simulink model "Silva_Simulink"  (R2024a)
settings: Solver=ode4  StartTime=0.0  StopTime=30  FixedStep=0.01  MaxStep=0.01  RelTol=1e-8  AbsTol=1e-8
values from neighbouring files (symbols this model uses):
  EA_0 = deg2rad([0 0 0]')    [Choi_SimulinkScript.m]    (also in SADS_UKF_Script.m = deg2rad([10 10 0]'); pointMassTest.m = [0 0 0]')
  J_0 = [1.815  -0.014 0.004 ... (first row only)    [Choi_SimulinkScript.m]    (also in Silva_SimulinkScript.m = [0.265 -0.014 -0.035; -0.014 0.246 -0.018; -0.035 -0.018 0.4; pointMassTest.m = diag([0.0226, 0.0257 0.0266]))
  kp = 0.5    [Silva_Matlab.m]    (also in Silva_Matlab_Implementation.m; Silva_SimulinkScript.m)
  m = 14.307    [Silva_Matlab.m]    (also in Silva_Matlab_Implementation.m; Silva_SimulinkScript.m; ukf.m)
  m_mmu = 2 * ((0.015*6) + (n*.236) + 0.177)    (= 2.894)    [Choi_SimulinkScript.m]    (also in Silva_Matlab.m = 0.7; Silva_Matlab_Implementation.m = 0.7; Silva_SimulinkScript.m = 0.7)
  omega_0 = [0 0.00 0.03]'    [Choi_SimulinkScript.m]    (also in SADS_UKF_Script.m = [0 0.00 0.00]'; Silva_SimulinkScript.m = [0 0 0.005]')
  q_0 = [0.99 -0.005 -0.063 -0.105]'    [Choi_SimulinkScript.m]    (also in SADS_UKF_Script.m = eul2quat(EA_0',"XYZ")'; Silva_SimulinkScript.m = [1 0 0 0]'; pointMassTest.m = [0 0 0 1]')
  r_b_0 = [-1 -3 -5]'*10^-3    [Silva_SimulinkScript.m]    (also in pointMassTest.m = [1 -0.9 -1.4]'.*1e-4)
  r_est_0 = [0 0 0]'    [Silva_SimulinkScript.m]
  Rcm = [y(8); y(9); y(10)]    [Silva_Matlab.m]    (also in Silva_Matlab_Implementation.m; eom_ukf.m = [0; 0; y(7)]; ukf.m = [0.1; -0.3; -5]*1e-3)
settings Model: Creator=cocmc  LastModifiedBy=cocmc

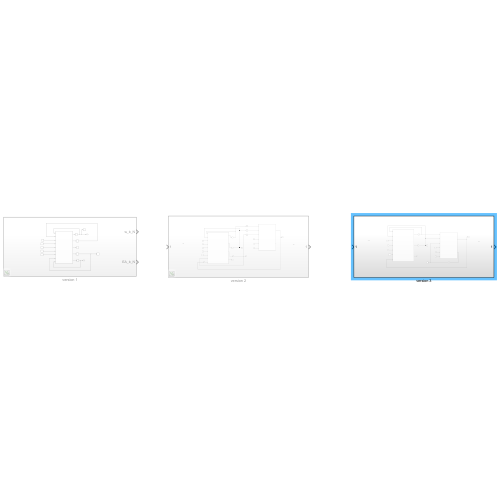
[thumbnail: Simulink's stored preview of the top-level diagram]
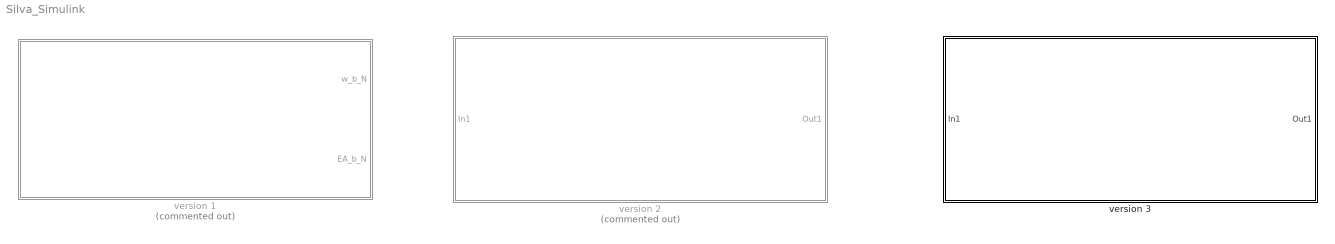
== system Silva_Simulink ==
  version 1 : Subsystem  Commented=on
  version 2 : Subsystem  Commented=on
  version 3 : Subsystem

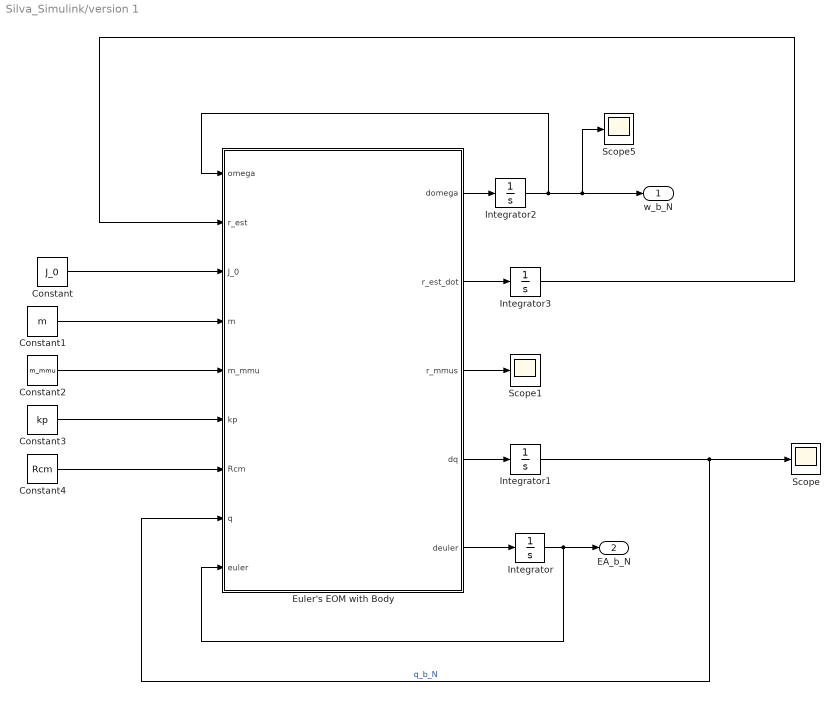
== system Silva_Simulink/version 1 ==
  Constant : Constant  Value=J_0
  Constant1 : Constant  Value=m
  Constant2 : Constant  Value=m_mmu
  Constant3 : Constant  Value=kp
  Constant4 : Constant  Value=Rcm
  Euler's EOM with Body : MATLAB Function  TreatAsAtomicUnit=on
  Integrator : Integrator  InitialCondition=EA_0
  Integrator1 : Integrator  InitialCondition=q_0
  Integrator2 : Integrator  InitialCondition=omega_0
  Integrator3 : Integrator  InitialCondition=r_est_0
  Scope : Scope
  Scope1 : Scope
  Scope5 : Scope
  w_b_N : Outport
  EA_b_N : Outport  Port=2
  wires:
  Constant1/1 -> Euler's EOM with Body/4(m)
  Euler's EOM with Body/1(domega) -> Integrator2/1
  Integrator2/1 -> Euler's EOM with Body/1(omega), Scope5/1, w_b_N/1
  Euler's EOM with Body/5(deuler) -> Integrator/1
  Integrator/1 -> EA_b_N/1, Euler's EOM with Body/9(euler)
  Euler's EOM with Body/4(dq) -> Integrator1/1
  Integrator1/1 -> Scope/1, Euler's EOM with Body/8(q)  "q_b_N"
  Euler's EOM with Body/2(r_est_dot) -> Integrator3/1
  Integrator3/1 -> Euler's EOM with Body/2(r_est)
  Constant/1 -> Euler's EOM with Body/3(J_0)
  Constant2/1 -> Euler's EOM with Body/5(m_mmu)
  Constant3/1 -> Euler's EOM with Body/6(kp)
  Constant4/1 -> Euler's EOM with Body/7(Rcm)
  Euler's EOM with Body/3(r_mmus) -> Scope1/1

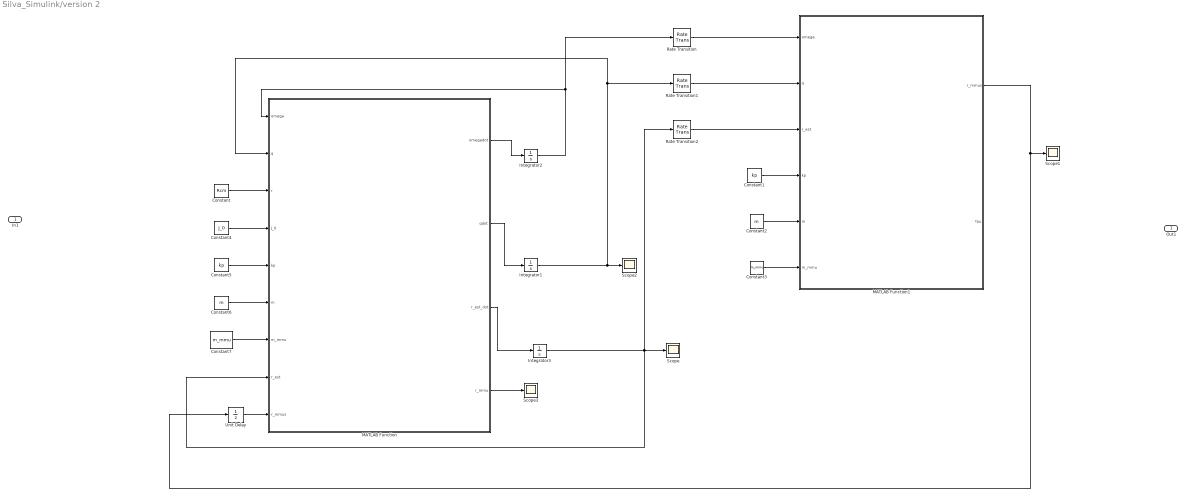
== system Silva_Simulink/version 2 ==
  In1 : Inport
  Constant : Constant  Value=Rcm
  Constant1 : Constant  Value=kp
  Constant2 : Constant  Value=m
  Constant3 : Constant  Value=m_mmu
  Constant4 : Constant  Value=J_0
  Constant5 : Constant  Value=kp
  Constant6 : Constant  Value=m
  Constant7 : Constant  Value=m_mmu
  Integrator1 : Integrator  InitialCondition=q_0
  Integrator2 : Integrator  InitialCondition=omega_0
  Integrator3 : Integrator  InitialCondition=r_est_0
  MATLAB Function : MATLAB Function  TreatAsAtomicUnit=on
  MATLAB Function1 : MATLAB Function  TreatAsAtomicUnit=on
  Rate Transition : RateTransition  InitialCondition=omega_0  OutPortSampleTime=control_sample
  Rate Transition1 : RateTransition  InitialCondition=q_0  OutPortSampleTime=control_sample
  Rate Transition2 : RateTransition  InitialCondition=r_est_0  OutPortSampleTime=control_sample
  Scope{,1..3} (4 alike) : Scope
  Unit Delay : UnitDelay  InitialCondition=[0 0 0]'  SampleTime=-1  HasFrameUpgradeWarning=on
  Out1 : Outport
  wires:
  MATLAB Function/1(omegadot) -> Integrator2/1
  MATLAB Function/2(qdot) -> Integrator1/1
  Integrator1/1 -> MATLAB Function/2(q), Rate Transition1/1, Scope2/1
  Integrator2/1 -> Rate Transition/1, MATLAB Function/1(omega)
  MATLAB Function/3(r_est_dot) -> Integrator3/1
  Integrator3/1 -> Rate Transition2/1, Scope/1, MATLAB Function/8(r_est)
  Constant/1 -> MATLAB Function/3(r)
  Constant1/1 -> MATLAB Function1/4(kp)
  MATLAB Function1/1(r_mmus) -> Unit Delay/1, Scope1/1
  Rate Transition/1 -> MATLAB Function1/1(omega)
  Rate Transition1/1 -> MATLAB Function1/2(q)
  Rate Transition2/1 -> MATLAB Function1/3(r_est)
  Unit Delay/1 -> MATLAB Function/9(r_mmus)
  Constant2/1 -> MATLAB Function1/5(m)
  Constant3/1 -> MATLAB Function1/6(m_mmu)
  Constant4/1 -> MATLAB Function/4(J_0)
  Constant5/1 -> MATLAB Function/5(kp)
  Constant6/1 -> MATLAB Function/6(m)
  Constant7/1 -> MATLAB Function/7(m_mmu)
  MATLAB Function/4(r_mmu) -> Scope3/1

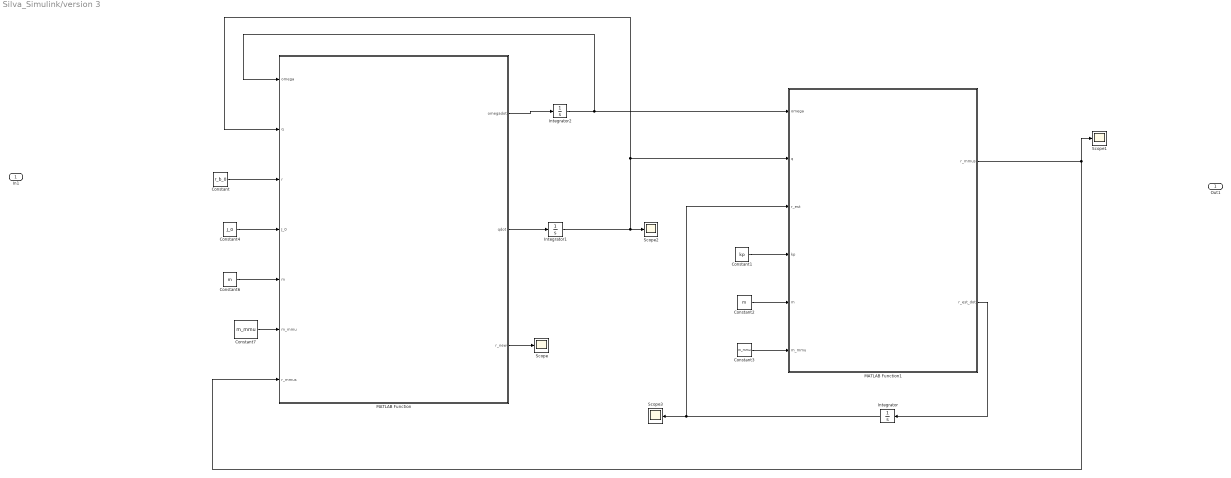
== system Silva_Simulink/version 3 ==
  In1 : Inport
  Constant : Constant  Value=r_b_0
  Constant1 : Constant  Value=kp
  Constant2 : Constant  Value=m
  Constant3 : Constant  Value=m_mmu
  Constant4 : Constant  Value=J_0
  Constant6 : Constant  Value=m
  Constant7 : Constant  Value=m_mmu
  Integrator : Integrator  InitialCondition=r_est_0
  Integrator1 : Integrator  InitialCondition=q_0
  Integrator2 : Integrator  InitialCondition=omega_0
  MATLAB Function : MATLAB Function  TreatAsAtomicUnit=on
  MATLAB Function1 : MATLAB Function  TreatAsAtomicUnit=on
  Scope{,1..3} (4 alike) : Scope
  Out1 : Outport
  wires:
  MATLAB Function/1(omegadot) -> Integrator2/1
  MATLAB Function/2(qdot) -> Integrator1/1
  Constant/1 -> MATLAB Function/3(r)
  Constant1/1 -> MATLAB Function1/4(kp)
  Constant2/1 -> MATLAB Function1/5(m)
  Constant3/1 -> MATLAB Function1/6(m_mmu)
  Constant4/1 -> MATLAB Function/4(J_0)
  Constant6/1 -> MATLAB Function/5(m)
  Constant7/1 -> MATLAB Function/6(m_mmu)
  MATLAB Function1/2(r_est_dot) -> Integrator/1
  Integrator/1 -> Scope3/1, MATLAB Function1/3(r_est)
  MATLAB Function/3(r_new) -> Scope/1
  MATLAB Function1/1(r_mmus) -> MATLAB Function/7(r_mmus), Scope1/1
  Integrator2/1 -> MATLAB Function1/1(omega), MATLAB Function/1(omega)
  Integrator1/1 -> MATLAB Function1/2(q), MATLAB Function/2(q), Scope2/1

== matlab function Silva_Simulink/version 3/MATLAB Function ==
  data: omega input; q input; r input; J_0 input; m input; m_mmu input; r_mmus input; omegadot output; qdot output; r_new output
function [omegadot, qdot,r_new] = fcn(omega,q,r,J_0,m,m_mmu,r_mmus)
% Equations of motion developed in the work of Chesi.

g = 9.81; % 


% Quaternion rates
qdot = 0.5*[0 -omega(1) -omega(2) -omega(3);
             omega(1) 0 omega(3) -omega(2);
             omega(2) -omega(3) 0 omega(1);
             omega(3) omega(2) -omega(1) 0]*q;

% Gravity vector in body-frame
Rbi = [2*q(1)^2-1+2*q(2)^2 2*q(2)*q(3)-2*q(1)*q(4) 2*q(2)*q(4)+2*q(1)*q(3);
       2*q(2)*q(3)+2*q(1)*q(4) 2*q(1)^2-1+2*q(3)^2 2*q(3)*q(4)-2*q(1)*q(2);
       2*q(2)*q(4)-2*q(1)*q(3) 2*q(3)*q(4)+2*q(1)*q(2) 2*q(1)^2-1+2*q(4)^2];

g_b = Rbi' * [0; 0; -9.81];

MMUx = [r_mmus(1); -0.22; 0];
MMUy = [0.22; r_mmus(2); 0];
MMUz = [-0.22; 0; r_mmus(3)];


Jaug = [m*(r(2)^2+r(3)^2) -m*r(1)*r(2) -m*r(1)*r(3);
        -m*r(1)*r(2) m*(r(1)^2+r(3)^2) -m*r(2)*r(3);
        -m*r(1)*r(3) -m*r(2)*r(3) m*(r(1)^2+r(2)^2)];

J = J_0 + Jaug;

% Update of inertia tensor
MMUxCross = [0 -MMUx(3) MMUx(2);
             MMUx(3) 0 -MMUx(1);
             -MMUx(2) MMUx(1) 0];

MMUyCross = [0 -MMUy(3) MMUy(2);
             MMUy(3) 0 -MMUy(1);
             -MMUy(2) MMUy(1) 0];

MMUzCross = [0 -MMUz(3) MMUz(2);
             MMUz(3) 0 -MMUz(1);
             -MMUz(2) MMUz(1) 0];

J = J - m_mmu * (MMUxCross*MMUxCross + MMUyCross*MMUyCross + MMUzCross*MMUzCross);

u = [1 0 0; % column vectors that each mass slides along
     0 1 0;
     0 0 1];



sum = zeros(size(u,2), 1);
for i = 1:size(u,2)
    sum = sum + m_mmu*r_mmus(i)*u(:,i);
end

r_new = r + (1/m).*sum;


tau = m_mmu * cross(r_mmus,g_b);
tau = 0;

r = r_new;

%% Dynamics equation
omegadot=J\(-cross(omega,J*omega)+cross(r,g_b*m)+tau);

== matlab function Silva_Simulink/version 3/MATLAB Function1 ==
  data: omega input; q input; r_mmus output; r_est_dot output; r_est input; kp input; m input; m_mmu input
function [r_mmus,r_est_dot] = fcn(omega,q,r_est,kp,m,m_mmu)
    Rbi = [2*q(1)^2-1+2*q(2)^2 2*q(2)*q(3)-2*q(1)*q(4) 2*q(2)*q(4)+2*q(1)*q(3);
           2*q(2)*q(3)+2*q(1)*q(4) 2*q(1)^2-1+2*q(3)^2 2*q(3)*q(4)-2*q(1)*q(2);
           2*q(2)*q(4)-2*q(1)*q(3) 2*q(3)*q(4)+2*q(1)*q(2) 2*q(1)^2-1+2*q(4)^2];

    g_b = Rbi' * [0; 0; -9.81];


    % Projection operator
    P = eye(3) - g_b*g_b'/norm(g_b)^2;
    omega_p = P*omega;
    gbcross = [0 -g_b(3) g_b(2);
               g_b(3) 0 -g_b(1);
              -g_b(2) g_b(1) 0];
    
    Phi = -m*gbcross;
    tau = -Phi*r_est-kp*omega_p;
    
    r_mmus = gbcross*tau/(norm(g_b)^2*m_mmu);


    % Adaptive control law for the estimated unbalance vector
    r_est_dot = Phi'*omega;

== matlab function Silva_Simulink/version 2/MATLAB Function1 ==
  data: omega input; q input; r_mmus output; r_est input; kp input; m input; m_mmu input; tau output
function [r_mmus,tau] = fcn(omega,q,r_est,kp,m,m_mmu)
    Rbi = [2*q(1)^2-1+2*q(2)^2 2*q(2)*q(3)-2*q(1)*q(4) 2*q(2)*q(4)+2*q(1)*q(3);
           2*q(2)*q(3)+2*q(1)*q(4) 2*q(1)^2-1+2*q(3)^2 2*q(3)*q(4)-2*q(1)*q(2);
           2*q(2)*q(4)-2*q(1)*q(3) 2*q(3)*q(4)+2*q(1)*q(2) 2*q(1)^2-1+2*q(4)^2];

    gb = Rbi' * [0; 0; -9.81];
    gbcross = [0 -gb(3) gb(2);
               gb(3) 0 -gb(1);
              -gb(2) gb(1) 0];

    % control torque at end of time step
    
    Phi = -m*gbcross;
    P = eye(3) - gb*gb'/norm(gb)^2;
    omegap = P*omega;
    tau = -Phi*r_est-kp*omegap;

    % Determine the new r_mmus vector. Dynamics of the MMUs are not considered,
    % which means r_mmus changes instantaneously
    r_mmus = gbcross*tau/(norm(gb)^2*m_mmu);

== matlab function Silva_Simulink/version 2/MATLAB Function ==
  data: omega input; q input; r input; J_0 input; kp input; m input; m_mmu input; r_est input; r_mmus input; omegadot output; qdot output; r_est_dot output; r_mmu output
function [omegadot, qdot, r_est_dot,r_mmu] = fcn(omega,q,r,J_0,kp,m,m_mmu,r_est,r_mmus)
% Equations of motion developed in the work of Chesi.

g = 9.81; % 


% Quaternion rates
qdot = 0.5*[0 -omega(1) -omega(2) -omega(3);
             omega(1) 0 omega(3) -omega(2);
             omega(2) -omega(3) 0 omega(1);
             omega(3) omega(2) -omega(1) 0]*q;

% Gravity vector in body-frame
Rbi = [2*q(1)^2-1+2*q(2)^2 2*q(2)*q(3)-2*q(1)*q(4) 2*q(2)*q(4)+2*q(1)*q(3);
       2*q(2)*q(3)+2*q(1)*q(4) 2*q(1)^2-1+2*q(3)^2 2*q(3)*q(4)-2*q(1)*q(2);
       2*q(2)*q(4)-2*q(1)*q(3) 2*q(3)*q(4)+2*q(1)*q(2) 2*q(1)^2-1+2*q(4)^2];

g_b = Rbi' * [0; 0; -g];

% Projection operator
P = eye(3) - g_b*g_b'/norm(g_b)^2;
omega_p = P*omega;
gbcross = [0 -g_b(3) g_b(2);
           g_b(3) 0 -g_b(1);
          -g_b(2) g_b(1) 0];

Phi = -m*gbcross;
tau = -Phi*r_est-kp*omega_p;

r_mmu = gbcross*tau/(norm(g_b)^2*m_mmu);
tau = m_mmu * cross(r_mmu,g_b);

% Adaptive control law for the estimated unbalance vector
r_est_dot = Phi'*omega;

MMUx = [r_mmus(1); -0.22; 0];
MMUy = [0.22; r_mmus(2); 0];
MMUz = [-0.22; 0; r_mmus(3)];


Jaug = [m*(r(2)^2+r(3)^2) -m*r(1)*r(2) -m*r(1)*r(3);
        -m*r(1)*r(2) m*(r(1)^2+r(3)^2) -m*r(2)*r(3);
        -m*r(1)*r(3) -m*r(2)*r(3) m*(r(1)^2+r(2)^2)];

J = J_0 + Jaug;

% Update of inertia tensor
MMUxCross = [0 -MMUx(3) MMUx(2);
             MMUx(3) 0 -MMUx(1);
             -MMUx(2) MMUx(1) 0];

MMUyCross = [0 -MMUy(3) MMUy(2);
             MMUy(3) 0 -MMUy(1);
             -MMUy(2) MMUy(1) 0];

MMUzCross = [0 -MMUz(3) MMUz(2);
             MMUz(3) 0 -MMUz(1);
             -MMUz(2) MMUz(1) 0];

J = J - m_mmu * (MMUxCross*MMUxCross + MMUyCross*MMUyCross + MMUzCross*MMUzCross);



%% Dynamics equation
omegadot=J\(-cross(omega,J*omega)+cross(r,g_b*m)+tau);

== matlab function Silva_Simulink/version 1/Euler's EOM with Body ==
  data: omega input; r_est input; J_0 input; m input; m_mmu input; kp input; Rcm input; q input; domega output; r_est_dot output; r_mmus output; euler input; dq output; deuler output
function [domega,r_est_dot,r_mmus,dq,deuler] = fcn(omega,r_est,J_0,m,m_mmu,kp,Rcm,q,euler)

Rbi = [2*q(1)^2-1+2*q(2)^2 2*q(2)*q(3)-2*q(1)*q(4) 2*q(2)*q(4)+2*q(1)*q(3);
       2*q(2)*q(3)+2*q(1)*q(4) 2*q(1)^2-1+2*q(3)^2 2*q(3)*q(4)-2*q(1)*q(2);
       2*q(2)*q(4)-2*q(1)*q(3) 2*q(3)*q(4)+2*q(1)*q(2) 2*q(1)^2-1+2*q(4)^2];

g_b = Rbi' * [0; 0; -9.81];

g_b_cross = [0 -g_b(3) g_b(2);
           g_b(3) 0 -g_b(1);
          -g_b(2) g_b(1) 0];

Phi = -m*g_b_cross;



P = eye(3) - g_b*g_b'/norm(g_b)^2;
omega_p = P*omega;
control_torque = -Phi*r_est-kp*omega_p;


r_mmus = g_b_cross*control_torque/(norm(g_b)^2*m_mmu);


% DERIVATIVES
r_est_dot = Phi'*omega;

omega_cross = [0        -omega(3) omega(2);
            omega(3)  0         -omega(1);
           -omega(2)  omega(1) 0 ];

Jaug = [m*(Rcm(2)^2+Rcm(3)^2) -m*Rcm(1)*Rcm(2) -m*Rcm(1)*Rcm(3);
        -m*Rcm(1)*Rcm(2) m*(Rcm(1)^2+Rcm(3)^2) -m*Rcm(2)*Rcm(3);
        -m*Rcm(1)*Rcm(3) -m*Rcm(2)*Rcm(3) m*(Rcm(1)^2+Rcm(2)^2)];
%Jaug=0;
J = J_0 + Jaug;

MMUx = [r_mmus(1); -0.22; 0];
MMUy = [0.22; r_mmus(2); 0];
MMUz = [-0.22; 0; r_mmus(3)];
% Update of inertia tensor
MMUxCross = [0 -MMUx(3) MMUx(2);
             MMUx(3) 0 -MMUx(1);
            -MMUx(2) MMUx(1) 0];

MMUyCross = [0 -MMUy(3) MMUy(2);
             MMUy(3) 0 -MMUy(1);
            -MMUy(2) MMUy(1) 0];

MMUzCross = [0 -MMUz(3) MMUz(2);
             MMUz(3) 0 -MMUz(1);
            -MMUz(2) MMUz(1) 0];

J = J - m_mmu * (MMUxCross*MMUxCross + MMUyCross*MMUyCross + MMUzCross*MMUzCross);

% equations of motion
domega = J\(-cross(omega,J*omega + cross(Rcm,g_b*m) + control_torque));

% propogating kinematics...
Phi = euler(1);
Theta = euler(2);
Psi = euler(3);

matrix = (1/cos(Theta)).*[cos(Theta) sin(Phi)*sin(Theta)  cos(Phi)*sin(Theta);
                              0          cos(Phi)*cos(Theta) -sin(Phi)*cos(Theta);
                              0          sin(Phi)             cos(Phi)];

product = matrix * omega;

dPhi = product(1);
dTheta = product(2);
dPsi = product(3);

deuler = [dPhi dTheta dPsi]';

dq = 0.5*[0 -omega(1) -omega(2) -omega(3);
             omega(1) 0 omega(3) -omega(2);
             omega(2) -omega(3) 0 omega(1);
             omega(3) omega(2) -omega(1) 0]*q;
